simulink model "differentiation_integration"  (R2019b)
settings: Solver=VariableStepAuto  StartTime=0.0  StopTime=10.0  RelTol=1e-3
values from neighbouring files (symbols this model uses):
  A = 3    [diff_int.m]
  F = 2    [diff_int.m]    (also in spring_damp.m = 1)
  I = 2.3    [battery_run.m]    (also in diff_int.m = 3)
  Ti = 0.5    [diff_int.m]
libraries: simulink x1
settings Model: Creator=dgander  LastModifiedBy=dgander

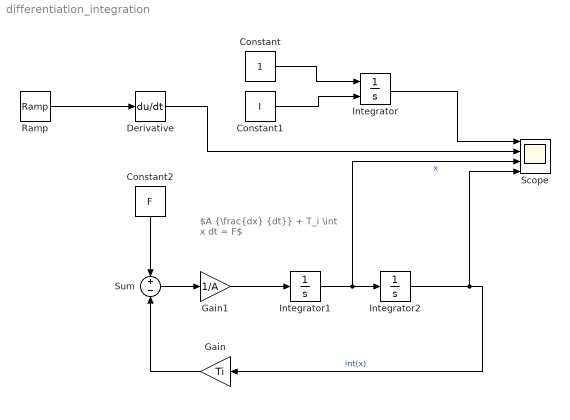
== system differentiation_integration ==
  note: $A {\frac{dx} {dt}} + T_i \int x dt = F$
  Constant : Constant
  Constant1 : Constant  Value=I
  Constant2 : Constant  Value=F
  Derivative : Derivative
  Gain : Gain  Gain=Ti
  Gain1 : Gain  Gain=1/A
  Integrator : Integrator  InitialConditionSource=external
  Integrator1 : Integrator
  Integrator2 : Integrator
  Ramp : simulink/Sources/Ramp  slope=1  start=0  InitialOutput=0
  Scope : Scope  NumInputPorts=4
  Sum : Sum  Inputs=+-
  wires:
  Constant/1 -> Integrator/1
  Integrator/1 -> Scope/1
  Derivative/1 -> Scope/2
  Ramp/1 -> Derivative/1
  Constant1/1 -> Integrator/2
  Integrator1/1 -> Scope/3, Integrator2/1  "x"
  Integrator2/1 -> Scope/4, Gain/1  "int(x)"
  Gain/1 -> Sum/2
  Sum/1 -> Gain1/1
  Gain1/1 -> Integrator1/1
  Constant2/1 -> Sum/1
